simulink model "Praktikum08Gruppe09"  (R2023b)
settings: Solver=VariableStepAuto  StartTime=0.0  StopTime=0.05  RelTol=1e-3
model workspace (MAT data in the model file):
  CodeRate = 0.75
  M = 16
  PunctureVector = [1; 1; 0; 1; 0; 1]
  TracebackDepth = 48
  Trelli : object (value not decoded)
  Ts = 5e-08
undefined symbols (not defined in the file): doppler, get, gray, hot, magnitude
libraries: dspstat3 x10, dspxfrm3 x8, dspobslib x7, commcnvcod2 x6, commdigbbndam3 x6, dspindex x6, commchan3 x4, commrflib2 x4, dspquant2 x4, commsink2 x4, dspsigops x4, commrandsrc3 x2
(part 2 of 2)

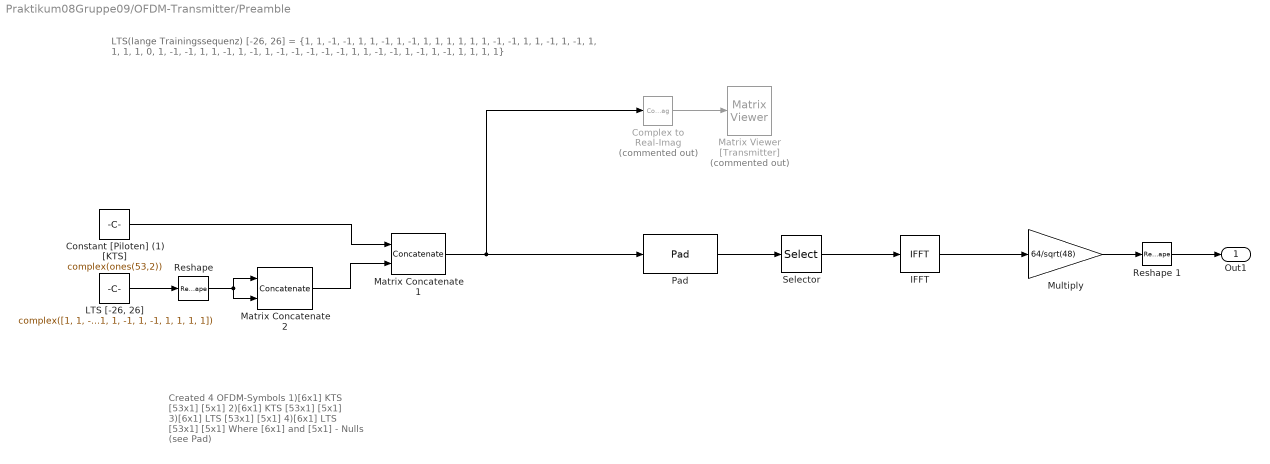
== system Praktikum08Gruppe09/OFDM-Transmitter/Preamble ==
  note: Created 4 OFDM-Symbols
      | 1)[6x1] KTS [53x1] [5x1]
      | 2)[6x1] KTS [53x1] [5x1]
      | 3)[6x1] LTS [53x1] [5x1]
      | 4)[6x1] LTS [53x1] [5x1]
      |
      | Where [6x1] and [5x1] - Nulls (see Pad)
  note: LTS(lange Trainingssequenz) [-26, 26] = {1, 1, -1, -1, 1, 1, -1, 1, -1, 1, 1, 1, 1, 1, 1, -1, -1, 1, 1, -1, 1, -1, 1, 1, 1, 1, 0, 1, -1, -1, 1, 1, -1, 1, -1, 1, -1, -1, -1, -1, -1, 1, 1, -1, -1, 1, -1, 1, -1, 1, 1, 1, 1}
  "Complex to Real-Imag " : ComplexToRealImag  Commented=on  Output=Real
  Constant [Piloten] (1) [KTS] : Constant  Value=complex(ones(53,2))  VectorParams1D=off
  "IFFT " : dspxfrm3/IFFT  FFTImplementation=Auto  CompMethod=Table lookup  TableOpt=NEW  TableOptActive=Speed  BitRevOrder=off  cs_in=off  Normalize=on  InheritFFTLength=on  FFTLength=64  WrapInput=on  mode=Complex  outSamplingMode=Sample based  roundingMode=Floor  overflowMode=off  firstCoeffDataTypeStr=Inherit: Same word length as input  firstCoeffLastDataTypeStr=Inherit: Same word length as input  outputMin=[]  outputMax=[]
  "LTS [-26, 26]" : Constant  Value=complex([1, 1, -1, -1, 1, 1, -1, 1, -1, 1, 1, 1, 1, 1, 1, -1, -1, 1, 1, -1, 1, -1, 1, 1, 1, 1, 0, 1, -1, -1, 1, 1, -1, 1, -1, 1, -1, -1, -1, -1, -1, 1, 1, -1, -1, 1, -1, 1, -1, 1, 1, 1, 1])  VectorParams1D=off
  Matrix Concatenate 1 : Concatenate  Mode=Multidimensional array  ConcatenateDimension=2
  Matrix Concatenate 2 : Concatenate  Mode=Multidimensional array  ConcatenateDimension=2
  Matrix Viewer [Transmitter] : dspobslib/Matrix Viewer  Commented=on  ImageParams=off  CMapStr=hot(256)  AxisColorbar=on  AxisParams=off  AxisOrigin=Upper left corner  AxisTickMode=User-defined  XTickRange=[1 4]  YTickRange=[1 53]  XLabel=X-axis  YLabel=Y-axis  ZLabel=Z-axis  FigPos=get(0,'defaultfigureposition')  AxisZoom=off
      settings: YMin=-1  YMax=1
  "Multiply " : Gain  Gain=64/sqrt(48)
  "Pad " : dspsigops/Pad  padAlong=Columns  dimsToPad=1  valSrc=Specify via dialog  padVal=0  spec=Output size  padNumOutRowsSpecMethod=User-specified  numOutRows=64  padNumOutColsSpecMethod=User-specified  numOutCols=1  isVarDimsMode=off  padBeginning=0  padEnd=0  outSizeMode=User-specified  outSize=1  padSigAt=End  trunc_flag=None  roundingMode=Floor  overflowMode=off  truncOrWrapMode=Truncate  wrap_flag=None
  "Reshape " : Reshape  OutputDimensionality=Column vector (2-D)
  Reshape 1 : Reshape  OutputDimensionality=Column vector (2-D)  OutputDimensions=[64,24]
  "Selector " : Selector  NumberOfDimensions=2  InputPortWidth=3  IndexOptions=Index vector (dialog),Select all  Indices=[27:64 1:26],1  OutputSizes=1,1
  Out1 : Outport
  wires:
  "Pad "/1 -> "Selector "/1
  "Selector "/1 -> "IFFT "/1
  "Multiply "/1 -> Reshape 1/1
  "IFFT "/1 -> "Multiply "/1
  Reshape 1/1 -> Out1/1
  Matrix Concatenate 1/1 -> "Pad "/1, "Complex to Real-Imag "/1
  "LTS [-26, 26]"/1 -> "Reshape "/1
  "Reshape "/1 -> Matrix Concatenate 2/2, Matrix Concatenate 2/1
  Matrix Concatenate 2/1 -> Matrix Concatenate 1/2
  Constant [Piloten] (1) [KTS]/1 -> Matrix Concatenate 1/1
  "Complex to Real-Imag "/1 -> Matrix Viewer [Transmitter]/1

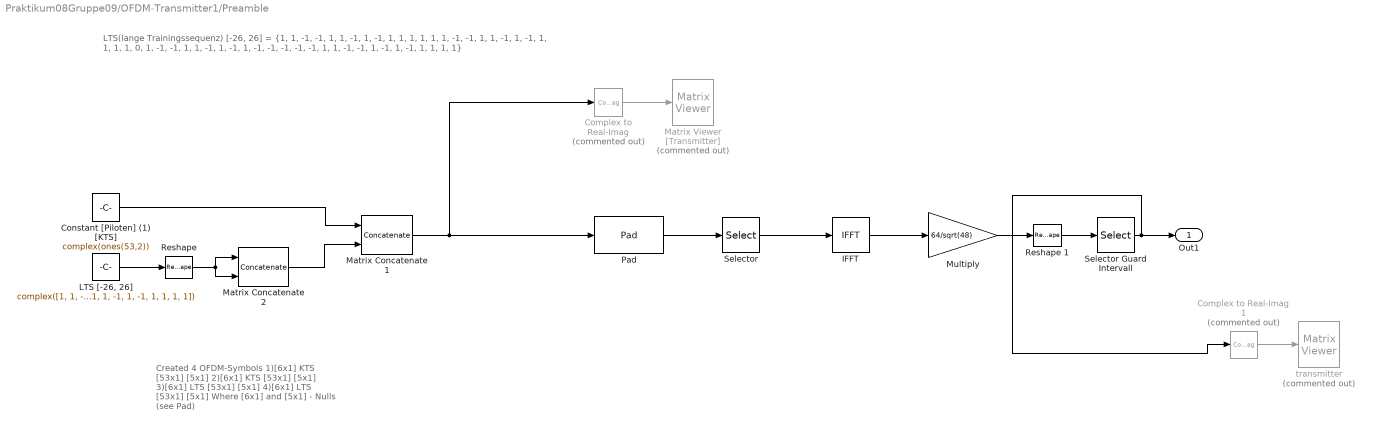
== system Praktikum08Gruppe09/OFDM-Transmitter1/Preamble ==
  note: Created 4 OFDM-Symbols
      | 1)[6x1] KTS [53x1] [5x1]
      | 2)[6x1] KTS [53x1] [5x1]
      | 3)[6x1] LTS [53x1] [5x1]
      | 4)[6x1] LTS [53x1] [5x1]
      |
      | Where [6x1] and [5x1] - Nulls (see Pad)
  note: LTS(lange Trainingssequenz) [-26, 26] = {1, 1, -1, -1, 1, 1, -1, 1, -1, 1, 1, 1, 1, 1, 1, -1, -1, 1, 1, -1, 1, -1, 1, 1, 1, 1, 0, 1, -1, -1, 1, 1, -1, 1, -1, 1, -1, -1, -1, -1, -1, 1, 1, -1, -1, 1, -1, 1, -1, 1, 1, 1, 1}
  "Complex to Real-Imag " : ComplexToRealImag  Commented=on  Output=Real
  Complex to Real-Imag 1 : ComplexToRealImag  Commented=on  Output=Real
  Constant [Piloten] (1) [KTS] : Constant  Value=complex(ones(53,2))  VectorParams1D=off
  "IFFT " : dspxfrm3/IFFT  FFTImplementation=Auto  CompMethod=Table lookup  TableOpt=NEW  TableOptActive=Speed  BitRevOrder=off  cs_in=off  Normalize=on  InheritFFTLength=on  FFTLength=64  WrapInput=on  mode=Complex  outSamplingMode=Sample based  roundingMode=Floor  overflowMode=off  firstCoeffDataTypeStr=Inherit: Same word length as input  firstCoeffLastDataTypeStr=Inherit: Same word length as input  outputMin=[]  outputMax=[]
  "LTS [-26, 26]" : Constant  Value=complex([1, 1, -1, -1, 1, 1, -1, 1, -1, 1, 1, 1, 1, 1, 1, -1, -1, 1, 1, -1, 1, -1, 1, 1, 1, 1, 0, 1, -1, -1, 1, 1, -1, 1, -1, 1, -1, -1, -1, -1, -1, 1, 1, -1, -1, 1, -1, 1, -1, 1, 1, 1, 1])  VectorParams1D=off
  Matrix Concatenate 1 : Concatenate  Mode=Multidimensional array  ConcatenateDimension=2
  Matrix Concatenate 2 : Concatenate  Mode=Multidimensional array  ConcatenateDimension=2
  Matrix Viewer [Transmitter] : dspobslib/Matrix Viewer  Commented=on  ImageParams=off  CMapStr=hot(256)  AxisColorbar=on  AxisParams=off  AxisOrigin=Upper left corner  AxisTickMode=User-defined  XTickRange=[1 4]  YTickRange=[1 53]  XLabel=X-axis  YLabel=Y-axis  ZLabel=Z-axis  FigPos=get(0,'defaultfigureposition')  AxisZoom=off
      settings: YMin=-1  YMax=1
  "Multiply " : Gain  Gain=64/sqrt(48)
  "Pad " : dspsigops/Pad  padAlong=Columns  dimsToPad=1  valSrc=Specify via dialog  padVal=0  spec=Output size  padNumOutRowsSpecMethod=User-specified  numOutRows=64  padNumOutColsSpecMethod=User-specified  numOutCols=1  isVarDimsMode=off  padBeginning=0  padEnd=0  outSizeMode=User-specified  outSize=1  padSigAt=End  trunc_flag=None  roundingMode=Floor  overflowMode=off  truncOrWrapMode=Truncate  wrap_flag=None
  "Reshape " : Reshape  OutputDimensionality=Column vector (2-D)
  Reshape 1 : Reshape  OutputDimensionality=Column vector (2-D)  OutputDimensions=[64,24]
  "Selector " : Selector  NumberOfDimensions=2  InputPortWidth=3  IndexOptions=Index vector (dialog),Select all  Indices=[27:64 1:26],1  OutputSizes=1,1
  Selector Guard Intervall : Selector  NumberOfDimensions=2  InputPortWidth=3  IndexOptions=Index vector (dialog),Select all  Indices=[33:64, 1:128, 225:256, 129:256],1  OutputSizes=1,1
  transmitter : dspobslib/Matrix Viewer  Commented=on  ImageParams=off  CMapStr=gray(256)  AxisColorbar=on  AxisParams=off  AxisOrigin=Upper left corner  AxisTickMode=Auto  XTickRange=[0 1]  YTickRange=[0 1]  XLabel=X-axis  YLabel=Y-axis  ZLabel=Z-axis  FigPos=get(0,'defaultfigureposition')  AxisZoom=off
      settings: YMin=-1.4434  YMax=7.6499
  Out1 : Outport
  wires:
  "Pad "/1 -> "Selector "/1
  "Selector "/1 -> "IFFT "/1
  Reshape 1/1 -> Selector Guard Intervall/1
  Matrix Concatenate 1/1 -> "Pad "/1, "Complex to Real-Imag "/1
  "LTS [-26, 26]"/1 -> "Reshape "/1
  "Reshape "/1 -> Matrix Concatenate 2/2, Matrix Concatenate 2/1
  Matrix Concatenate 2/1 -> Matrix Concatenate 1/2
  Constant [Piloten] (1) [KTS]/1 -> Matrix Concatenate 1/1
  "Complex to Real-Imag "/1 -> Matrix Viewer [Transmitter]/1
  "IFFT "/1 -> "Multiply "/1
  "Multiply "/1 -> Reshape 1/1
  Complex to Real-Imag 1/1 -> transmitter/1
  Selector Guard Intervall/1 -> Complex to Real-Imag 1/1, Out1/1
